simulink model "Continuous_Hybrid_Systems"  (R2022a)
settings: Solver=ode45  StartTime=0.0  StopTime=10  RelTol=1e-3
settings Model: Creator=csamak  LastModifiedBy=csamak

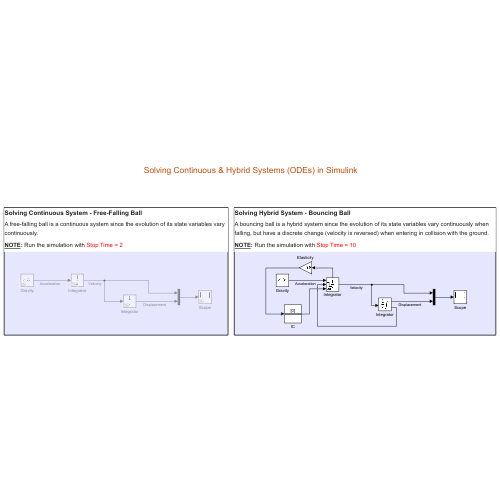
[thumbnail: Simulink's stored preview of the top-level diagram]
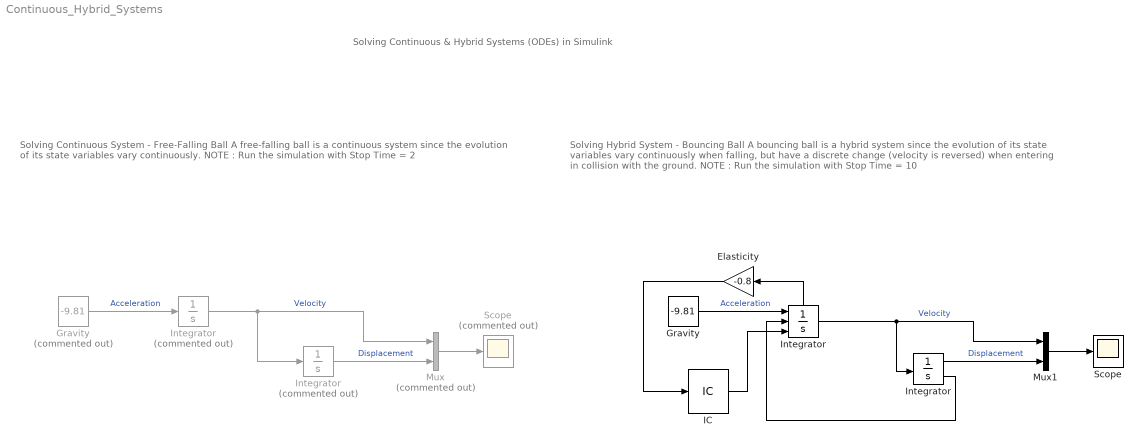
== system Continuous_Hybrid_Systems ==
  note: Solving Continuous & Hybrid Systems (ODEs) in Simulink
  note: Solving Continuous System - Free-Falling Ball
      | A free-falling ball is a continuous system since the evolution of its state variables vary continuously.
      | NOTE : Run the simulation with Stop Time = 2
  note: Solving Hybrid System - Bouncing Ball
      | A bouncing ball is a hybrid system since the evolution of its state variables vary continuously when falling, but have a discrete change (velocity is reversed) when entering in collision with the ground.
      | NOTE : Run the simulation with Stop Time = 10
  "   Integrator   " : Integrator  InitialCondition=15  LimitOutput=on  LowerSaturationLimit=0  ShowSaturationPort=on
  "  Integrator  " : Integrator  ExternalReset=falling  InitialConditionSource=external  ShowStatePort=on
  " Gravity " : Constant  Value=-9.81
  " Integrator " : Integrator  Commented=on  InitialCondition=15
  " Scope " : Scope
  Elasticity : Gain  Gain=-0.8
  Gravity : Constant  Commented=on  Value=-9.81
  IC : InitialCondition  Value=0
  Integrator : Integrator  Commented=on
  Mux : Mux  Commented=on  Inputs=2
  Mux1 : Mux  Inputs=2
  Scope : Scope  Commented=on
  wires:
  Gravity/1 -> Integrator/1  "Acceleration"
  Integrator/1 -> Mux/1, " Integrator "/1  "Velocity"
  " Integrator "/1 -> Mux/2  "Displacement"
  Mux/1 -> Scope/1
  " Gravity "/1 -> "  Integrator  "/1  "Acceleration"
  "  Integrator  "/1 -> Mux1/1, "   Integrator   "/1  "Velocity"
  "   Integrator   "/1 -> Mux1/2  "Displacement"
  Mux1/1 -> " Scope "/1
  "   Integrator   "/2 -> "  Integrator  "/2
  "  Integrator  "/State -> Elasticity/1
  Elasticity/1 -> IC/1
  IC/1 -> "  Integrator  "/3
